simulink model "cooling_model"  (R2022a)
settings: Solver=VariableStepAuto  StartTime=4192  StopTime=20000  RelTol=1e-3
values from neighbouring files (symbols this model uses):
  area_air_fan = (fan_qty*pi.*fan_dia^2)./4'    [Cooling_Script.m]
  area_fins = n_fins * (h_fin-delta_fin) * w_radiator * 2    [Cooling_Script.m]
  area_fins_inverter = n_fins_inverter * (h_fin_inverter-delta_fin_inverter) * w_radiator_inverter * 2    [Cooling_Script.m]
  area_fins_motor = n_fins_motor * (h_fin_motor-delta_fin_motor) * w_radiator_motor * 2    [Cooling_Script.m]
  area_primary = 2 * L_tube * w_radiator * (n_fin_rows) - 2 * delta_fin * w_radiator * n_fins + 2 * h_fin * w_radiator * n_fin_rows + 2 * h_tube * n_tubes * L_tube    [Cooling_Script.m]
  area_primary_inverter = 2 * L_tube_inverter * w_radiator_inverter * (n_fin_rows_inverter) - 2 * delta_fin_inverter * w_radiator_inverter * n_fins_inverter + 2 * h_fin_inverter * w_radiator_inverter * n_fin_rows_inverter + 2 * h_tube_inverter * n_tubes_inverter * L_tube_inverter    [Cooling_Script.m]
  area_primary_motor = 2 * L_tube_motor * w_radiator_motor * (n_fin_rows_motor) - 2 * delta_fin_motor * w_radiator_motor * n_fins_motor + 2 * h_fin_motor * w_radiator_motor * n_fin_rows_motor + 2 * h_tube_motor * n_tubes_motor * L_tube_motor    [Cooling_Script.m]
  cp_air = 1004    [Cooling_Script.m]
  h_tube = 0.0015    [Cooling_Script.m]
  h_tube_inverter = 0.0015    [Cooling_Script.m]
  h_tube_motor = 0.0015    [Cooling_Script.m]
  HC_min = 10    [Cooling_Script.m]
  HC_nom = 100    [Cooling_Script.m]
  L_tube = 46*25.4./1000    [Cooling_Script.m]
  L_tube_inverter = 46*25.4./1000    [Cooling_Script.m]
  L_tube_motor = 46*25.4./1000    [Cooling_Script.m]
  n_tubes = 36    [Cooling_Script.m]
  n_tubes_inverter = 36    [Cooling_Script.m]
  n_tubes_motor = 36    [Cooling_Script.m]
  rho_air = 1.2    [Cooling_Script.m]
  vel_air_nom = 1    [Cooling_Script.m]
  w_radiator = 2.6*25.4    (= 66.04)    [Cooling_Script.m]
  w_radiator_inverter = 2.6*25.4    (= 66.04)    [Cooling_Script.m]
  w_radiator_motor = 2.6*25.4    (= 66.04)    [Cooling_Script.m]
libraries: fl_lib x65, nesl_utility x35, SimscapeFluids_lib x12, aerolibconvert2 x9
(part 1 of 2)
settings Model: PacingRate=7  Creator=saumilj  LastModifiedBy=saumilj

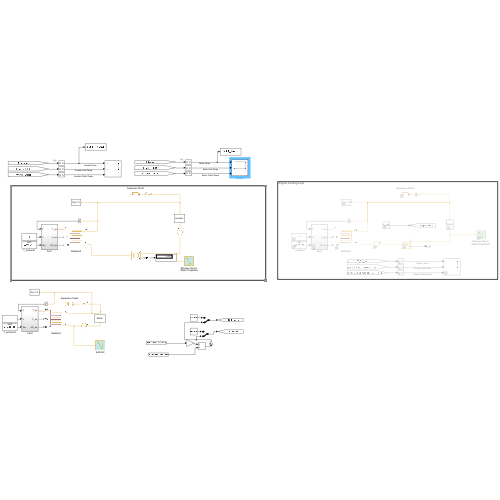
[thumbnail: Simulink's stored preview of the top-level diagram]
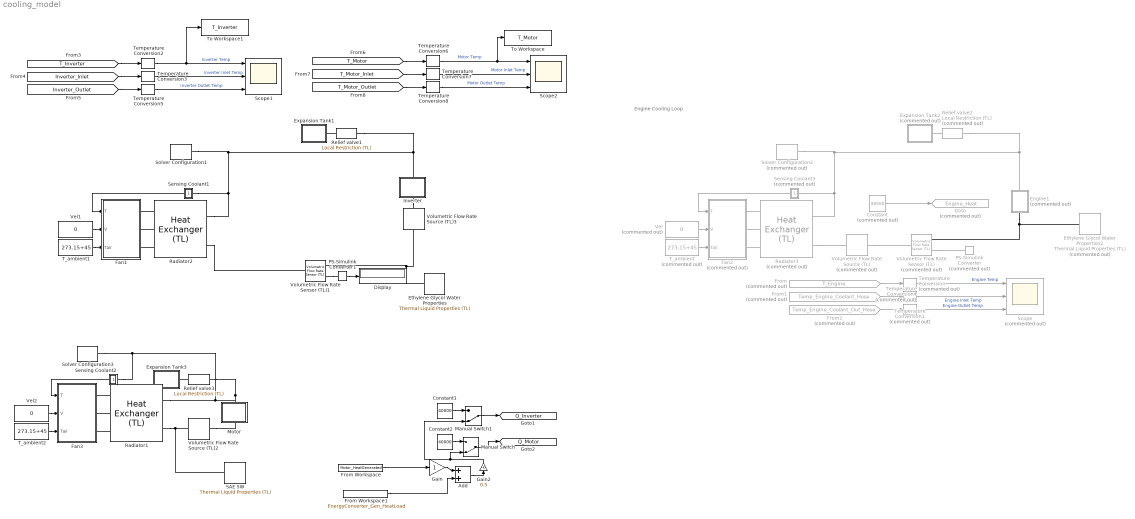
== system cooling_model ==
  note: Engine Cooling Loop
  Add : Sum
  Constant : Constant  Commented=on  Value=80000
  Constant1 : Constant  Value=40000
  Constant2 : Constant  Value=40000
  Display : Display
  Engine1 : Subsystem  Tag=PublishSubsystem  Commented=on
      settings: PortSchema="{\"entries\":[{\"content\":{\"sides\":[{\"content\":{\"connectorIds\":[]},\"type\":\"ConnectorPlacement.EquallySpacedRectSide\",\"uuid\":\"ac213905-571d-4802-86f4-209dcc725585\"},{\"content\":{\"connectorIds\":[],\"side\":\"RIGHT\"},\"type\":\"ConnectorPlacement.EquallySpacedRectSide\",\"uuid\":\"d2c48898-fea5-4b13-99f1-692c4ae7991e\"},{\"content\":{\"connectorIds\":[\"LConn1\"],\"side\":\"TOP\"},\"type\":\"ConnectorPlacement.EquallySpacedRectSide\",\"uuid\":\"96c2b262-82b5-4793-b4c5-6a92a22b5fd9\"},{\"content\":{\"connectorIds\":[\"RConn1\"],\"side\":\"BOTTOM\"},\"type\":\"ConnectorPlacement.EquallySpacedRectSide\",\"uuid\":\"b403586d-fe60-4930-b0ca-7a9e68811f94\"}]},\"type\":\"ConnectorPlacement.EquallySpacedConnector\",\"uuid\":\"afb30120-f19b-44b2-997c-30915d066b29\"}],\"packageUris\":[\"http://schema.mathworks.com/mf0/Connector/R2020b\"],\"version\":\"1.0\"}"
      mask Display: disp(get_param(gcb, 'Name'))
  Ethylene Glycol Water Properties : SimscapeFluids_lib/Thermal Liquid/Utilities/Thermal Liquid Properties (TL)  fluid_list=3  concentration_param_EG=1  concentration_param_PG=1  c_mass_SW=3.5e-3  c_mass_EG=0.1  c_mass_PG=0.1  c_mass_GL=0.1  c_vol_EG=0.5  c_vol_PG=0.1  beta_const_EG=2.1791 GPa  beta_const_PG=2.1791 GPa  beta_const_GL=2.1791 GPa  p_min_EG=0.01 MPa  p_min_PG=0.01 MPa  p_min_GL=0.01 MPa  p_max_EG=50 MPa  p_max_PG=50 MPa  p_max_GL=50 MPa  p_atm=0.101325 MPa
      settings: SourceProductBaseCode=SH
  Ethylene Glycol Water Properties2 : SimscapeFluids_lib/Thermal Liquid/Utilities/Thermal Liquid Properties (TL)  Commented=on  fluid_list=3  concentration_param_EG=1  concentration_param_PG=1  c_mass_SW=3.5e-3  c_mass_EG=0.1  c_mass_PG=0.1  c_mass_GL=0.1  c_vol_EG=0.5  c_vol_PG=0.1  beta_const_EG=2.1791 GPa  beta_const_PG=2.1791 GPa  beta_const_GL=2.1791 GPa  p_min_EG=0.01 MPa  p_min_PG=0.01 MPa  p_min_GL=0.01 MPa  p_max_EG=50 MPa  p_max_PG=50 MPa  p_max_GL=50 MPa  p_atm=0.101325 MPa
      settings: SourceProductBaseCode=SH
  Expansion Tank1 : Subsystem
      mask Display: image('sscfluids_engine_cooling_system_expansion_tank_image.png')
  Expansion Tank2 : Subsystem  Commented=on
      mask Display: image('sscfluids_engine_cooling_system_expansion_tank_image.png')
  Expansion Tank3 : Subsystem
      mask Display: image('sscfluids_engine_cooling_system_expansion_tank_image.png')
  Fan1 : Subsystem
  Fan2 : Subsystem  Commented=on
  Fan3 : Subsystem
  From : From  Commented=on  GotoTag=T_Engine  TagVisibility=global
  From Workspace : FromWorkspace  VariableName=Motor_HeatGenerated
  From Workspace1 : FromWorkspace  VariableName=EnergyConverter_Gen_HeatLoad
  From1 : From  Commented=on  GotoTag=Temp_Engine_Coolant_Hose  TagVisibility=global
  From2 : From  Commented=on  GotoTag=Temp_Engine_Coolant_Out_Hose  TagVisibility=global
  Gain : Gain
  Gain2 : Gain  Gain=0.5
  Goto : Goto  Commented=on  GotoTag=Engine_Heat  TagVisibility=global
  Inverter : Subsystem  Tag=PublishSubsystem
      settings: PortSchema="{\"entries\":[{\"content\":{\"sides\":[{\"content\":{\"connectorIds\":[]},\"type\":\"ConnectorPlacement.EquallySpacedRectSide\",\"uuid\":\"ac213905-571d-4802-86f4-209dcc725585\"},{\"content\":{\"connectorIds\":[],\"side\":\"RIGHT\"},\"type\":\"ConnectorPlacement.EquallySpacedRectSide\",\"uuid\":\"d2c48898-fea5-4b13-99f1-692c4ae7991e\"},{\"content\":{\"connectorIds\":[\"LConn1\"],\"side\":\"TOP\"},\"type\":\"ConnectorPlacement.EquallySpacedRectSide\",\"uuid\":\"96c2b262-82b5-4793-b4c5-6a92a22b5fd9\"},{\"content\":{\"connectorIds\":[\"RConn1\"],\"side\":\"BOTTOM\"},\"type\":\"ConnectorPlacement.EquallySpacedRectSide\",\"uuid\":\"b403586d-fe60-4930-b0ca-7a9e68811f94\"}]},\"type\":\"ConnectorPlacement.EquallySpacedConnector\",\"uuid\":\"afb30120-f19b-44b2-997c-30915d066b29\"}],\"packageUris\":[\"http://schema.mathworks.com/mf0/Connector/R2020b\"],\"version\":\"1.0\"}"
      mask Display: disp(get_param(gcb, 'Name'))
  Manual Switch : ManualSwitch  CurrentSetting=0
  Manual Switch1 : ManualSwitch  CurrentSetting=0
  Motor : Subsystem  Tag=PublishSubsystem
      settings: PortSchema="{\"entries\":[{\"content\":{\"sides\":[{\"content\":{\"connectorIds\":[]},\"type\":\"ConnectorPlacement.EquallySpacedRectSide\",\"uuid\":\"ac213905-571d-4802-86f4-209dcc725585\"},{\"content\":{\"connectorIds\":[],\"side\":\"RIGHT\"},\"type\":\"ConnectorPlacement.EquallySpacedRectSide\",\"uuid\":\"d2c48898-fea5-4b13-99f1-692c4ae7991e\"},{\"content\":{\"connectorIds\":[\"LConn1\"],\"side\":\"TOP\"},\"type\":\"ConnectorPlacement.EquallySpacedRectSide\",\"uuid\":\"96c2b262-82b5-4793-b4c5-6a92a22b5fd9\"},{\"content\":{\"connectorIds\":[\"RConn1\"],\"side\":\"BOTTOM\"},\"type\":\"ConnectorPlacement.EquallySpacedRectSide\",\"uuid\":\"b403586d-fe60-4930-b0ca-7a9e68811f94\"}]},\"type\":\"ConnectorPlacement.EquallySpacedConnector\",\"uuid\":\"afb30120-f19b-44b2-997c-30915d066b29\"}],\"packageUris\":[\"http://schema.mathworks.com/mf0/Connector/R2020b\"],\"version\":\"1.0\"}"
      mask Display: disp(get_param(gcb, 'Name'))
  PS-Simulink Converter : nesl_utility/PS-Simulink Converter  Commented=on  PhysicalDomain=network_engine_domain  SubClassName=ps_output  LeftPortType=input  RightPortType=output  PseudoPeriodic=off  Frequencies=[]  VectorFormat=inherit  Unit=inherit  AffineConversion=off
      settings: SourceProductBaseCode=SS,PW,VE
  PS-Simulink Converter1 : nesl_utility/PS-Simulink Converter  PhysicalDomain=network_engine_domain  SubClassName=ps_output  LeftPortType=input  RightPortType=output  PseudoPeriodic=off  Frequencies=[]  VectorFormat=inherit  Unit=inherit  AffineConversion=off
      settings: SourceProductBaseCode=SS,PW,VE
  Radiator1 : SimscapeFluids_lib/Fluid Network Interfaces/Heat Exchangers/Heat Exchanger (TL)  hex_type=fluids.interfaces.enum.flow_arrangement_spec.parallel_counter  shell_num=1  cross_type=4  NTU_TLU=[0.5, 1.0, 2.0, 3.0, 4.0, 5.0]  CR_TLU=[0.0, 0.25, 0.5, 0.75, 1.0]  eff_TLU=[0.3, 0.3, 0.3, 0.3, 0.3; 0.6, 0.55, 0.5, 0.47, 0.43; 0.85, 0.76, 0.68, 0.61, 0.55; 0.94, 0.83, 0.72, 0.65, 0.58; 0.98, 0.86, 0.75, 0.66, 0.58; 0.99, 0.86, 0.75, 0.66, 0.58]  R_wall=0.014/(381*n_tubes_motor*w_radiator_motor*L_tube_motor) K/W  min_flow_area_1=n_tubes_motor*(w_radiator_motor*h_tube_motor) m^2  Dh_press_1=4*(w_radiator_motor*h_tube_motor)/(2 * (w_radiator_motor+h_tube_motor)) m  liquid_volume_1=n_tubes_motor*(w_radiator_motor*h_tube_motor)*L_tube_motor m^3  Re_lam_1=2000  Re_tur_1=4000  pressure_loss_spec_1=2  pressure_loss_coeff_1=15  length_press_1=L_tube_motor m  length_add_1=0.1 m  roughness_1=15e-6 m  Re_friction_TLU_1=[400.0, 1000.0, 1500.0, 3000.0, 4000.0, 6000.0, 10000.0, 20000.0, 40000.0, 60000.0, 100000.0, 100000000.0]  friction_factor_TLU_1=[0.264, 0.112, 0.071, 0.0417, 0.0387, 0.0268, 0.025, 0.0232, 0.0226, 0.022, 0.0214, 0.0214]  shape_factor_1=64  Re_Euler_TLU_1=[50.0, 500.0, 1000.0, 2000.0]  Euler_TLU_1=[4.4505, 0.6864, 0.4791, 0.3755]  heat_transfer_spec_1=2  heat_transfer_area_1=n_tubes_motor*2*(L_tube_motor*w_radiator_motor+L_tube_motor*h_tube_motor) m^2  heat_coeff_1=2000 W/(m^2 * K)  length_heat_1=L_tube_motor m  Nu_lam_1=3.66  Re_Colburn_TLU_1=[100.0, 150.0, 1000.0]  Colburn_factor_TLU_1=[0.019, 0.013, 0.002]  Re_Nu_TLU_1=[100.0, 150.0, 1000.0]  Pr_Nu_TLU_1=[1.0, 10.0]  Nu_TLU_1=[3.72, 4.21; 3.75, 4.44; 4.21, 7.15]  fouling_factor_1=0 m^2*K/W  min_heat_coeff_1=5 W/(m^2 * K)  heat_transfer_area_2=area_primary_motor+area_fins_motor m^2  fouling_factor_2=0 m^2*K/W  min_heat_coeff_2=0.01 W/(m^2 * K)  dynamic_compressibility_1=1  T0_1=293.15+25 K  p0_1=0.101325 MPa  mdot1_TLU=[.1, .2] kg/s  mdot2_TLU=[.2, .3] kg/s  SD_TLU=[35, 35; 50, 50] kW/K  Q_check=1  mdot_dp_TLU_1=[.1, .2] kg/s  p_diff_TLU_1=[.003, .005] MPa  T_ref_in_1=293.15 K  p_ref_in_1=0.101325 MPa  mdot_threshold_1=1e-3 kg/s  area_1=0.01 m^2
      settings: SourceProductBaseCode=SH  InternalSimscapePortConfiguration="{\"Bottom\":[],\"Left\":[{\"id\":\"A1\",\"label\":\"A1\",\"type\":\"foundation.thermal_liquid.thermal_liquid\"},{\"id\":\"B1\",\"label\":\"B1\",\"type\":\"foundation.thermal_liquid.thermal_liquid\"}],\"Right\":[{\"id\":\"H2\",\"label\":\"H2\",\"type\":\"foundation.thermal.thermal\"},{\"id\":\"C2\",\"label\":\"C2\",\"type\":\"input\"},{\"id\":\"HC2\",\"label\":\"HC2\",\"type\":\"input\"}],\"Top\":[]}"
  Radiator2 : SimscapeFluids_lib/Fluid Network Interfaces/Heat Exchangers/Heat Exchanger (TL)  hex_type=fluids.interfaces.enum.flow_arrangement_spec.parallel_counter  shell_num=1  cross_type=4  NTU_TLU=[0.5, 1.0, 2.0, 3.0, 4.0, 5.0]  CR_TLU=[0.0, 0.25, 0.5, 0.75, 1.0]  eff_TLU=[0.3, 0.3, 0.3, 0.3, 0.3; 0.6, 0.55, 0.5, 0.47, 0.43; 0.85, 0.76, 0.68, 0.61, 0.55; 0.94, 0.83, 0.72, 0.65, 0.58; 0.98, 0.86, 0.75, 0.66, 0.58; 0.99, 0.86, 0.75, 0.66, 0.58]  R_wall=0.014/(381*n_tubes_inverter*w_radiator_inverter*L_tube_inverter) K/W  min_flow_area_1=n_tubes_inverter*(w_radiator_inverter*h_tube_inverter) m^2  Dh_press_1=4*(w_radiator_inverter*h_tube_inverter)/(2 * (w_radiator_inverter+h_tube_inverter)) m  liquid_volume_1=n_tubes_inverter*(w_radiator_inverter*h_tube_inverter)*L_tube_inverter m^3  Re_lam_1=2000  Re_tur_1=4000  pressure_loss_spec_1=2  pressure_loss_coeff_1=15  length_press_1=L_tube_inverter m  length_add_1=0.1 m  roughness_1=15e-6 m  Re_friction_TLU_1=[400.0, 1000.0, 1500.0, 3000.0, 4000.0, 6000.0, 10000.0, 20000.0, 40000.0, 60000.0, 100000.0, 100000000.0]  friction_factor_TLU_1=[0.264, 0.112, 0.071, 0.0417, 0.0387, 0.0268, 0.025, 0.0232, 0.0226, 0.022, 0.0214, 0.0214]  shape_factor_1=64  Re_Euler_TLU_1=[50.0, 500.0, 1000.0, 2000.0]  Euler_TLU_1=[4.4505, 0.6864, 0.4791, 0.3755]  heat_transfer_spec_1=2  heat_transfer_area_1=n_tubes_inverter*2*(L_tube_inverter*w_radiator_inverter+L_tube_inverter*h_tube_inverter) m^2  heat_coeff_1=2000 W/(m^2 * K)  length_heat_1=L_tube_inverter m  Nu_lam_1=3.66  Re_Colburn_TLU_1=[100.0, 150.0, 1000.0]  Colburn_factor_TLU_1=[0.019, 0.013, 0.002]  Re_Nu_TLU_1=[100.0, 150.0, 1000.0]  Pr_Nu_TLU_1=[1.0, 10.0]  Nu_TLU_1=[3.72, 4.21; 3.75, 4.44; 4.21, 7.15]  fouling_factor_1=0 m^2*K/W  min_heat_coeff_1=5 W/(m^2 * K)  heat_transfer_area_2=area_primary_inverter+area_fins_inverter m^2  fouling_factor_2=0 m^2*K/W  min_heat_coeff_2=0.01 W/(m^2 * K)  dynamic_compressibility_1=1  T0_1=293.15+25 K  p0_1=0.101325 MPa  mdot1_TLU=[.1, .2] kg/s  mdot2_TLU=[.2, .3] kg/s  SD_TLU=[35, 35; 50, 50] kW/K  Q_check=1  mdot_dp_TLU_1=[.1, .2] kg/s  p_diff_TLU_1=[.003, .005] MPa  T_ref_in_1=293.15 K  p_ref_in_1=0.101325 MPa  mdot_threshold_1=1e-3 kg/s  area_1=0.01 m^2
      settings: SourceProductBaseCode=SH  InternalSimscapePortConfiguration="{\"Bottom\":[],\"Left\":[{\"id\":\"A1\",\"label\":\"A1\",\"type\":\"foundation.thermal_liquid.thermal_liquid\"},{\"id\":\"B1\",\"label\":\"B1\",\"type\":\"foundation.thermal_liquid.thermal_liquid\"}],\"Right\":[{\"id\":\"H2\",\"label\":\"H2\",\"type\":\"foundation.thermal.thermal\"},{\"id\":\"C2\",\"label\":\"C2\",\"type\":\"input\"},{\"id\":\"HC2\",\"label\":\"HC2\",\"type\":\"input\"}],\"Top\":[]}"
  Radiator3 : SimscapeFluids_lib/Fluid Network Interfaces/Heat Exchangers/Heat Exchanger (TL)  Commented=on  hex_type=fluids.interfaces.enum.flow_arrangement_spec.parallel_counter  shell_num=1  cross_type=4  NTU_TLU=[0.5, 1.0, 2.0, 3.0, 4.0, 5.0]  CR_TLU=[0.0, 0.25, 0.5, 0.75, 1.0]  eff_TLU=[0.3, 0.3, 0.3, 0.3, 0.3; 0.6, 0.55, 0.5, 0.47, 0.43; 0.85, 0.76, 0.68, 0.61, 0.55; 0.94, 0.83, 0.72, 0.65, 0.58; 0.98, 0.86, 0.75, 0.66, 0.58; 0.99, 0.86, 0.75, 0.66, 0.58]  R_wall=0.014/(381*n_tubes*w_radiator*L_tube) K/W  min_flow_area_1=n_tubes*(w_radiator*h_tube) m^2  Dh_press_1=4*(w_radiator*h_tube)/(2 * (w_radiator+h_tube)) m  liquid_volume_1=n_tubes*(w_radiator*h_tube)*L_tube m^3  Re_lam_1=2000  Re_tur_1=4000  pressure_loss_spec_1=2  pressure_loss_coeff_1=15  length_press_1=L_tube m  length_add_1=0.1 m  roughness_1=15e-6 m  Re_friction_TLU_1=[400.0, 1000.0, 1500.0, 3000.0, 4000.0, 6000.0, 10000.0, 20000.0, 40000.0, 60000.0, 100000.0, 100000000.0]  friction_factor_TLU_1=[0.264, 0.112, 0.071, 0.0417, 0.0387, 0.0268, 0.025, 0.0232, 0.0226, 0.022, 0.0214, 0.0214]  shape_factor_1=64  Re_Euler_TLU_1=[50.0, 500.0, 1000.0, 2000.0]  Euler_TLU_1=[4.4505, 0.6864, 0.4791, 0.3755]  heat_transfer_spec_1=2  heat_transfer_area_1=n_tubes*2*(L_tube*w_radiator+L_tube*h_tube) m^2  heat_coeff_1=2000 W/(m^2 * K)  length_heat_1=L_tube m  Nu_lam_1=3.66  Re_Colburn_TLU_1=[100.0, 150.0, 1000.0]  Colburn_factor_TLU_1=[0.019, 0.013, 0.002]  Re_Nu_TLU_1=[100.0, 150.0, 1000.0]  Pr_Nu_TLU_1=[1.0, 10.0]  Nu_TLU_1=[3.72, 4.21; 3.75, 4.44; 4.21, 7.15]  fouling_factor_1=0 m^2*K/W  min_heat_coeff_1=5 W/(m^2 * K)  heat_transfer_area_2=area_primary+area_fins m^2  fouling_factor_2=0 m^2*K/W  min_heat_coeff_2=0.01 W/(m^2 * K)  dynamic_compressibility_1=1  T0_1=293.15 K  p0_1=0.101325 MPa  mdot1_TLU=[.1, .2] kg/s  mdot2_TLU=[.2, .3] kg/s  SD_TLU=[35, 35; 50, 50] kW/K  Q_check=1  mdot_dp_TLU_1=[.1, .2] kg/s  p_diff_TLU_1=[.003, .005] MPa  T_ref_in_1=293.15 K  p_ref_in_1=0.101325 MPa  mdot_threshold_1=1e-3 kg/s  area_1=0.01 m^2
      settings: SourceProductBaseCode=SH  InternalSimscapePortConfiguration="{\"Bottom\":[],\"Left\":[{\"id\":\"A1\",\"label\":\"A1\",\"type\":\"foundation.thermal_liquid.thermal_liquid\"},{\"id\":\"B1\",\"label\":\"B1\",\"type\":\"foundation.thermal_liquid.thermal_liquid\"}],\"Right\":[{\"id\":\"H2\",\"label\":\"H2\",\"type\":\"foundation.thermal.thermal\"},{\"id\":\"C2\",\"label\":\"C2\",\"type\":\"input\"},{\"id\":\"HC2\",\"label\":\"HC2\",\"type\":\"input\"}],\"Top\":[]}"
  Relief valve1 : fl_lib/Thermal Liquid/Elements/Local Restriction (TL)  restriction_type=foundation.enum.restriction_type.fixed  restriction_area=pi*0.005^2 m^2  min_area=1e-10 m^2  max_area=0.005 m^2  area=pi*0.01^2 m^2  Cd=0.7  pressure_recovery=1  Re_c=12
      settings: SourceProductBaseCode=PW,SS,VE
  Relief valve2 : fl_lib/Thermal Liquid/Elements/Local Restriction (TL)  Commented=on  restriction_type=foundation.enum.restriction_type.fixed  restriction_area=pi*0.005^2 m^2  min_area=1e-10 m^2  max_area=0.005 m^2  area=pi*0.01^2 m^2  Cd=0.7  pressure_recovery=1  Re_c=12
      settings: SourceProductBaseCode=PW,SS,VE
  Relief valve3 : fl_lib/Thermal Liquid/Elements/Local Restriction (TL)  restriction_type=foundation.enum.restriction_type.fixed  restriction_area=pi*0.005^2 m^2  min_area=1e-10 m^2  max_area=0.005 m^2  area=pi*0.01^2 m^2  Cd=0.7  pressure_recovery=1  Re_c=12
      settings: SourceProductBaseCode=PW,SS,VE
  SAE 5W : SimscapeFluids_lib/Thermal Liquid/Utilities/Thermal Liquid Properties (TL)  fluid_list=fluids.thermal_liquid.utilities.enum.thermal_liquid_fluid_list.sae5w30  concentration_param_EG=1  concentration_param_PG=1  c_mass_SW=3.5e-3  c_mass_EG=0.1  c_mass_PG=0.1  c_mass_GL=0.1  c_vol_EG=0.5  c_vol_PG=0.1  beta_const_EG=2.1791 GPa  beta_const_PG=2.1791 GPa  beta_const_GL=2.1791 GPa  p_min_EG=0.01 MPa  p_min_PG=0.01 MPa  p_min_GL=0.01 MPa  p_max_EG=50 MPa  p_max_PG=50 MPa  p_max_GL=50 MPa  p_atm=0.101325 MPa
      settings: SourceProductBaseCode=SH
  Scope : Scope  Commented=on  NumInputPorts=3
  Scope1 : Scope  NumInputPorts=3
  Scope2 : Scope  NumInputPorts=3
  Sensing Coolant1 : Subsystem
      mask Display: disp('T');
  Sensing Coolant2 : Subsystem
      mask Display: disp('T');
  Sensing Coolant3 : Subsystem  Commented=on
      mask Display: disp('T');
  Solver Configuration1 : nesl_utility/Solver Configuration  PhysicalDomain=network_engine_domain  SubClassName=solver  LeftPortType=input  RightPortType=generic  Tones=[]  Harmonics=[]  SimulateNoise=off  Profile=off  UseLocalSampling=off  EnableSwitchedLinearOptims=on  FrequencyDomain=off  UseCCode=off  RelTol=0.001  AbsTol=1e-06  MinStep=1e-09  ToWorkspace=off  RevertToSquareIcSolve=off  NumHomotopyIterations=100  PhasorMode=off  PhasorModeNumHarmonics=1  IndexReductionMethod=DerivativeReplacement  DoDC=off  ResidualTolerance=1e-09  UseLocalSolver=off  LocalSolverChoice=NE_BACKWARD_EULER_ADVANCER  LocalSolverSampleTime=0.001  DoFixedCost=off  MaxNonlinIter=3  MaxModeIter=2  ComputeImpulses=off  ImpulseIterations=2  LinearAlgebra=auto  LinearAlgebraNumThread=0  EquationFormulation=NE_TIME_EF  DelaysMemoryBudget=1024  AutomaticFiltering=on  FilteringTimeConstant=0.001  PartitionStorageMethod=AS_NEEDED  PartitionMemoryBudget=1024  PartitionMethod=ROBUST
      settings: SourceProductBaseCode=SS,PW,VE
  Solver Configuration2 : nesl_utility/Solver Configuration  Commented=on  PhysicalDomain=network_engine_domain  SubClassName=solver  LeftPortType=input  RightPortType=generic  Tones=[]  Harmonics=[]  SimulateNoise=off  Profile=off  UseLocalSampling=off  EnableSwitchedLinearOptims=on  FrequencyDomain=off  UseCCode=off  RelTol=0.001  AbsTol=1e-06  MinStep=1e-09  ToWorkspace=off  RevertToSquareIcSolve=off  NumHomotopyIterations=100  PhasorMode=off  PhasorModeNumHarmonics=1  IndexReductionMethod=DerivativeReplacement  DoDC=off  ResidualTolerance=1e-09  UseLocalSolver=off  LocalSolverChoice=NE_BACKWARD_EULER_ADVANCER  LocalSolverSampleTime=0.001  DoFixedCost=off  MaxNonlinIter=3  MaxModeIter=2  ComputeImpulses=off  ImpulseIterations=2  LinearAlgebra=auto  LinearAlgebraNumThread=0  EquationFormulation=NE_TIME_EF  DelaysMemoryBudget=1024  AutomaticFiltering=on  FilteringTimeConstant=0.001  PartitionStorageMethod=AS_NEEDED  PartitionMemoryBudget=1024  PartitionMethod=ROBUST
      settings: SourceProductBaseCode=SS,PW,VE
  Solver Configuration3 : nesl_utility/Solver Configuration  PhysicalDomain=network_engine_domain  SubClassName=solver  LeftPortType=input  RightPortType=generic  Tones=[]  Harmonics=[]  SimulateNoise=off  Profile=off  UseLocalSampling=off  EnableSwitchedLinearOptims=on  FrequencyDomain=off  UseCCode=off  RelTol=0.001  AbsTol=1e-06  MinStep=1e-09  ToWorkspace=off  RevertToSquareIcSolve=off  NumHomotopyIterations=100  PhasorMode=off  PhasorModeNumHarmonics=1  IndexReductionMethod=DerivativeReplacement  DoDC=off  ResidualTolerance=1e-09  UseLocalSolver=off  LocalSolverChoice=NE_BACKWARD_EULER_ADVANCER  LocalSolverSampleTime=0.001  DoFixedCost=off  MaxNonlinIter=3  MaxModeIter=2  ComputeImpulses=off  ImpulseIterations=2  LinearAlgebra=auto  LinearAlgebraNumThread=0  EquationFormulation=NE_TIME_EF  DelaysMemoryBudget=1024  AutomaticFiltering=on  FilteringTimeConstant=0.001  PartitionStorageMethod=AS_NEEDED  PartitionMemoryBudget=1024  PartitionMethod=ROBUST
      settings: SourceProductBaseCode=SS,PW,VE
  T_ambient : Constant  Commented=on  Value=273.15+45
  T_ambient1 : Constant  Value=273.15+45
  T_ambient2 : Constant  Value=273.15+45
  Temperature Conversion : aerolibconvert2/Temperature Conversion  Commented=on  IU=K  OU=C
      settings: SourceProductBaseCode=AE
  Temperature Conversion1 : aerolibconvert2/Temperature Conversion  Commented=on  IU=K  OU=C
      settings: SourceProductBaseCode=AE
  Temperature Conversion{2..3,5..8} (6 alike) : aerolibconvert2/Temperature Conversion  IU=K  OU=C
      settings: SourceProductBaseCode=AE
  Temperature Conversion4 : aerolibconvert2/Temperature Conversion  Commented=on  IU=K  OU=C
      settings: SourceProductBaseCode=AE
  To Workspace : ToWorkspace  VariableName=T_Motor  SaveFormat=Timeseries  SampleTime=-1
  To Workspace1 : ToWorkspace  VariableName=T_Inverter  SaveFormat=Timeseries  SampleTime=-1
  Vel : Constant  Commented=on  Value=0
  Vel1 : Constant  Value=0
  Vel2 : Constant  Value=0
  Volumetric Flow Rate Sensor (TL) : fl_lib/Thermal Liquid/Sensors/Volumetric Flow Rate Sensor (TL)  Commented=on
      settings: SourceProductBaseCode=PW,SS,VE  InternalSimscapePortConfiguration="{\"Bottom\":[],\"Left\":[{\"id\":\"A\",\"label\":\"A\",\"type\":\"foundation.thermal_liquid.thermal_liquid\"}],\"Right\":[{\"id\":\"B\",\"label\":\"B\",\"type\":\"foundation.thermal_liquid.thermal_liquid\"},{\"id\":\"V\",\"label\":\"V\",\"type\":\"output\"}],\"Top\":[]}"
  Volumetric Flow Rate Sensor (TL)1 : fl_lib/Thermal Liquid/Sensors/Volumetric Flow Rate Sensor (TL)
      settings: SourceProductBaseCode=PW,SS,VE  InternalSimscapePortConfiguration="{\"Bottom\":[],\"Left\":[{\"id\":\"A\",\"label\":\"A\",\"type\":\"foundation.thermal_liquid.thermal_liquid\"}],\"Right\":[{\"id\":\"B\",\"label\":\"B\",\"type\":\"foundation.thermal_liquid.thermal_liquid\"},{\"id\":\"V\",\"label\":\"V\",\"type\":\"output\"}],\"Top\":[]}"
  Volumetric Flow Rate Source (TL) : fl_lib/Thermal Liquid/Sources/Volumetric Flow Rate Source (TL)  Commented=on  commanded_volumetric_flow=60 lpm  area=0.01 m^2
      settings: SourceProductBaseCode=PW,SS,VE  InternalSimscapePortConfiguration="{\"Bottom\":[],\"Left\":[{\"id\":\"A\",\"label\":\"A\",\"type\":\"foundation.thermal_liquid.thermal_liquid\"}],\"Right\":[{\"id\":\"B\",\"label\":\"B\",\"type\":\"foundation.thermal_liquid.thermal_liquid\"}],\"Top\":[]}"
  Volumetric Flow Rate Source (TL)2 : fl_lib/Thermal Liquid/Sources/Volumetric Flow Rate Source (TL)  commanded_volumetric_flow=20*6 lpm  area=0.01 m^2
      settings: SourceProductBaseCode=PW,SS,VE  InternalSimscapePortConfiguration="{\"Bottom\":[],\"Left\":[{\"id\":\"A\",\"label\":\"A\",\"type\":\"foundation.thermal_liquid.thermal_liquid\"}],\"Right\":[{\"id\":\"B\",\"label\":\"B\",\"type\":\"foundation.thermal_liquid.thermal_liquid\"}],\"Top\":[]}"
  Volumetric Flow Rate Source (TL)3 : fl_lib/Thermal Liquid/Sources/Volumetric Flow Rate Source (TL)  commanded_volumetric_flow=60 lpm  area=0.01 m^2
      settings: SourceProductBaseCode=PW,SS,VE  InternalSimscapePortConfiguration="{\"Bottom\":[],\"Left\":[{\"id\":\"A\",\"label\":\"A\",\"type\":\"foundation.thermal_liquid.thermal_liquid\"}],\"Right\":[{\"id\":\"B\",\"label\":\"B\",\"type\":\"foundation.thermal_liquid.thermal_liquid\"}],\"Top\":[]}"
  tag scope: Q_Inverter=global, Q_Motor=global
  wires:
  Constant/1 -> Goto/1
  Sensing Coolant3/1(Out1) -> Fan2/1(T)
  T_ambient/1 -> Fan2/3(Tair)
  Vel/1 -> Fan2/2(V)
  From/1 -> Temperature Conversion/1
  From1/1 -> Temperature Conversion1/1
  From2/1 -> Temperature Conversion4/1
  Temperature Conversion/1 -> Scope/1  "Engine Temp"
  Temperature Conversion1/1 -> Scope/2  "Engine Inlet Temp"
  Temperature Conversion4/1 -> Scope/3  "Engine Outlet Temp"
  Temperature Conversion5/1 -> Scope1/3  "Inverter Outlet Temp"
  Temperature Conversion3/1 -> Scope1/2  "Inverter Inlet Temp"
  Temperature Conversion2/1 -> To Workspace1/1, Scope1/1  "Inverter Temp"
  [Inverter_Outlet] -> Temperature Conversion5/1
  [Inverter_Inlet] -> Temperature Conversion3/1
  [T_Inverter] -> Temperature Conversion2/1
  Vel1/1 -> Fan1/2(V)
  T_ambient1/1 -> Fan1/3(Tair)
  Sensing Coolant1/1(Out1) -> Fan1/1(T)
  [T_Motor] -> Temperature Conversion6/1
  [T_Motor_Inlet] -> Temperature Conversion7/1
  [T_Motor_Outlet] -> Temperature Conversion8/1
  Temperature Conversion6/1 -> To Workspace/1, Scope2/1  "Motor Temp"
  Temperature Conversion7/1 -> Scope2/2  "Motor Inlet Temp"
  Temperature Conversion8/1 -> Scope2/3  "Motor Outlet Temp"
  Constant2/1 -> Manual Switch/1
  Manual Switch/1 -> [Q_Motor]
  PS-Simulink Converter1/1 -> Display/1
  Vel2/1 -> Fan3/2(V)
  Sensing Coolant2/1(Out1) -> Fan3/1(T)
  T_ambient2/1 -> Fan3/3(Tair)
  Constant1/1 -> Manual Switch1/1
  Manual Switch1/1 -> [Q_Inverter]
  From Workspace/1 -> Gain/1
  Gain/1 -> Add/1
  From Workspace1/1 -> Add/2
  Add/1 -> Gain2/1
  Gain2/1 -> Manual Switch1/2, Manual Switch/2
  connections:
  Volumetric Flow Rate Source (TL)/RConn1 -- Volumetric Flow Rate Sensor (TL)/LConn1
  Volumetric Flow Rate Sensor (TL)/RConn2 -- PS-Simulink Converter/LConn1
  Volumetric Flow Rate Sensor (TL)/RConn1 -- Ethylene Glycol Water Properties2/RConn1 -- Engine1/RConn1
  Relief valve2/LConn1 -- Expansion Tank2/RConn1
  Radiator3/RConn1 -- Fan2/RConn1
  Radiator3/RConn2 -- Fan2/RConn2
  Radiator3/RConn3 -- Fan2/RConn3
  Solver Configuration2/RConn1 -- Engine1/LConn1 -- Relief valve2/RConn1 -- Sensing Coolant3/LConn1 -- Radiator3/LConn1
  Radiator3/LConn2 -- Volumetric Flow Rate Source (TL)/LConn1
  Inverter/LConn1 -- Relief valve1/RConn1 -- Solver Configuration1/RConn1 -- Radiator2/LConn1 -- Sensing Coolant1/LConn1
  Radiator2/RConn3 -- Fan1/RConn3
  Radiator2/RConn2 -- Fan1/RConn2
  Radiator2/RConn1 -- Fan1/RConn1
  Relief valve1/LConn1 -- Expansion Tank1/RConn1
  Radiator2/LConn2 -- Volumetric Flow Rate Sensor (TL)1/LConn1
  Ethylene Glycol Water Properties/RConn1 -- Volumetric Flow Rate Source (TL)3/LConn1 -- Volumetric Flow Rate Sensor (TL)1/RConn1
  Inverter/RConn1 -- Volumetric Flow Rate Source (TL)3/RConn1
  Volumetric Flow Rate Sensor (TL)1/RConn2 -- PS-Simulink Converter1/LConn1
  SAE 5W/RConn1 -- Radiator1/LConn2 -- Volumetric Flow Rate Source (TL)2/LConn1
  Relief valve3/RConn1 -- Radiator1/LConn1 -- Solver Configuration3/RConn1 -- Sensing Coolant2/LConn1 -- Motor/LConn1
  Volumetric Flow Rate Source (TL)2/RConn1 -- Motor/RConn1
  Relief valve3/LConn1 -- Expansion Tank3/RConn1
  Radiator1/RConn1 -- Fan3/RConn1
  Radiator1/RConn2 -- Fan3/RConn2
  Radiator1/RConn3 -- Fan3/RConn3

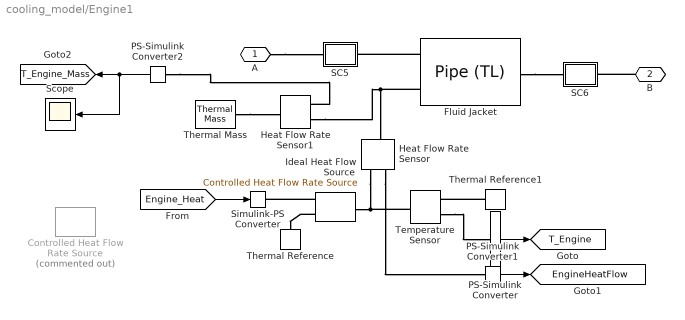
== system cooling_model/Engine1 ==
  Controlled Heat Flow Rate Source : fl_lib/Thermal/Thermal Sources/Controlled Heat Flow Rate Source  Commented=on
      settings: SourceProductBaseCode=PW,SS,VE
  Fluid Jacket : SimscapeFluids_lib/Thermal Liquid/Pipes & Fittings/Pipe (TL)  dynamic_compressibility=simscape.enum.onoff.off  inertia=simscape.enum.onoff.off  num_segments=1  pipe_length=0.2 m  area=pi*0.01^2 m^2  wall_spec=fluids.thermal_liquid.pipes_fittings.enum.wall_spec.rigid  Dh=0.005 m  wall_compliance=1.2e-6 m/MPa  wall_time_constant=0.01 s  elevation_spec=foundation.enum.constant_variable.constant  elevation_gain=0 m  g=9.81 m/s^2  pressure_loss_spec=fluids.thermal_liquid.pipes_fittings.enum.PressureLossSpec.Nominal  local_pressure_loss_spec=fluids.thermal_liquid.pipes_fittings.enum.LocalLossSpec.AggregateLength  length_add=0 m  loss_coefficient=0.1  roughness=1.5e-60 m  Re_friction_TLU=[ 400 1000 1.5e+3 3e+3 4e+3 6e+3 1e+4 2e+4 4e+4 6e+4 1e+5 1e+8 ]  friction_factor_TLU=[ 0.264 0.112 0.07099999999999999 0.0417 0.0387 0.0268 0.025 0.0232 0.0226 0.022 0.0214 0.0214 ]  shape_factor=1e-50  Re_lam=2e+3  Re_tur=4e+3  mdot_nominal=[ 0.1 1000 ] kg/s  p_diff_nominal=[ 0.00000001 0.000000001 ] MPa  mdot_threshold=1e-6 kg/s  heat_transfer_spec=fluids.thermal_liquid.pipes_fittings.enum.HeatTransferSpec.TabulatedNusselt  mdot_nominal_heat=[ 0.1 1 ] kg/s  T_in_nominal=[ 293.15 293.15 ] K  T_out_nominal=[ 300 300 ] K  p_in_nominal_heat=[ 0.101325 0.101325 ] MPa  T_wall_nominal=[ 303.15 303.15 ] K  a_coeff=0.023  b_Re_power=0.8  c_Pr_power=0.4  Nu_lam=3.66  Re_Colburn_TLU=[ 100 150 1000 ]  Colburn_factor_TLU=[ 0.019 0.013 0.002 ]  Re_Nu_TLU=Re_TLU  Pr_Nu_TLU=Pr_TLU  Nu_TLU=Nu_TLU  T0_vec=303.15 K  p0_vec=0.101325 MPa  mdot0=0.1 kg/s
      settings: SourceProductBaseCode=SH
  Heat Flow Rate Sensor : fl_lib/Thermal/Thermal Sensors/Heat Flow Rate Sensor
      settings: SourceProductBaseCode=PW,SS,VE
  Heat Flow Rate Sensor1 : fl_lib/Thermal/Thermal Sensors/Heat Flow Rate Sensor
      settings: SourceProductBaseCode=PW,SS,VE
  Ideal Heat Flow Source : fl_lib/Thermal/Thermal Sources/Controlled Heat Flow Rate Source
      settings: SourceProductBaseCode=PW,SS,VE
  PS-Simulink Converter : nesl_utility/PS-Simulink Converter  PhysicalDomain=network_engine_domain  SubClassName=ps_output  LeftPortType=input  RightPortType=output  PseudoPeriodic=off  Frequencies=[]  VectorFormat=1-D array  Unit=degC  AffineConversion=on
      settings: SourceProductBaseCode=SS,PW,VE
  PS-Simulink Converter1 : nesl_utility/PS-Simulink Converter  PhysicalDomain=network_engine_domain  SubClassName=ps_output  LeftPortType=input  RightPortType=output  PseudoPeriodic=off  Frequencies=[]  VectorFormat=inherit  Unit=inherit  AffineConversion=off
      settings: SourceProductBaseCode=SS,PW,VE
  PS-Simulink Converter2 : nesl_utility/PS-Simulink Converter  PhysicalDomain=network_engine_domain  SubClassName=ps_output  LeftPortType=input  RightPortType=output  PseudoPeriodic=off  Frequencies=[]  VectorFormat=inherit  Unit=inherit  AffineConversion=off
      settings: SourceProductBaseCode=SS,PW,VE
  SC5 : Subsystem
      mask Display: disp(get_param(gcb, 'Name'))
  SC6 : Subsystem
      mask Display: disp(get_param(gcb, 'Name'))
  Scope : Scope
  Simulink-PS Converter : nesl_utility/Simulink-PS Converter  PhysicalDomain=network_engine_domain  SubClassName=ps_input  LeftPortType=input  RightPortType=output  PseudoPeriodic=off  Frequencies=[]  NoiseDistribution=none  NoiseParameters=[]  Unit=W  AffineConversion=off  FilteringAndDerivatives=provide  SimscapeFilterOrder=1  InputFilterTimeConstant=0.001  UdotUserProvided=0
      settings: SourceProductBaseCode=SS,PW,VE
  Temperature Sensor : fl_lib/Thermal/Thermal Sensors/Temperature Sensor
      settings: SourceProductBaseCode=PW,SS,VE
  Thermal Mass : fl_lib/Thermal/Thermal Elements/Thermal Mass  mass=100 kg  sp_heat=447 J/(K*kg)  T_specify=on  T_priority=High  T=273+45 K  T_nominal_specify=off  T_nominal_unit=K  T_nominal_value=1  Q_specify=off  Q_priority=None  Q=0 W  Q_nominal_specify=off  Q_nominal_unit=W  Q_nominal_value=1
      settings: SourceProductBaseCode=PW,SS,VE
  Thermal Reference : fl_lib/Thermal/Thermal Elements/Thermal Reference
      settings: SourceProductBaseCode=PW,SS,VE
  Thermal Reference1 : fl_lib/Thermal/Thermal Elements/Thermal Reference
      settings: SourceProductBaseCode=PW,SS,VE
  A : PMIOPort  Side=Left
  B : PMIOPort  Port=2  Side=Right
  tag scope: EngineHeatFlow=global, T_Engine=global, T_Engine_Mass=global
  wires:
  [Engine_Heat] -> Simulink-PS Converter/1
  PS-Simulink Converter/1 -> [T_Engine]
  PS-Simulink Converter1/1 -> [EngineHeatFlow]
  PS-Simulink Converter2/1 -> Scope/1, [T_Engine_Mass]
  connections:
  Temperature Sensor/LConn1 -- Heat Flow Rate Sensor/RConn2 -- Ideal Heat Flow Source/LConn1
  B/RConn1 -- SC6/RConn1
  Ideal Heat Flow Source/RConn2 -- Thermal Reference/LConn1
  A/RConn1 -- SC5/LConn1
  Ideal Heat Flow Source/RConn1 -- Simulink-PS Converter/RConn1
  Thermal Reference1/LConn1 -- Temperature Sensor/RConn1
  Temperature Sensor/RConn2 -- PS-Simulink Converter/LConn1
  Fluid Jacket/LConn2 -- Heat Flow Rate Sensor1/RConn2 -- Heat Flow Rate Sensor/LConn1
  Heat Flow Rate Sensor/RConn1 -- PS-Simulink Converter1/LConn1
  Fluid Jacket/LConn1 -- SC5/RConn1
  Fluid Jacket/RConn1 -- SC6/LConn1
  PS-Simulink Converter2/LConn1 -- Heat Flow Rate Sensor1/RConn1
  Thermal Mass/LConn1 -- Heat Flow Rate Sensor1/LConn1

== system cooling_model/Expansion Tank1 ==
  Expansion Tank : SimscapeFluids_lib/Thermal Liquid/Tanks & Accumulators/Gas-Charged Accumulator (TL)  capacity=0.005 m^3  dead_volume=1e-5 m^3  p_precharge_gauge=0 MPa  k_sh=1.4  area=pi*0.01^2 m^2  stiff_coeff=1e6 MPa/m^3  damping_coeff=1e6 s*MPa/m^6  liquid_volume_specify=on  liquid_volume_priority=High  liquid_volume=1e-6 m^3  liquid_volume_nominal_specify=off  liquid_volume_nominal_unit=m^3  liquid_volume_nominal_value=1  liquid_mass_specify=off  liquid_mass_priority=None  liquid_mass=5 kg  liquid_mass_nominal_specify=off  liquid_mass_nominal_unit=kg  liquid_mass_nominal_value=1  p_accumulator_specify=off  p_accumulator_priority=High  p_accumulator=0.101325 MPa  p_accumulator_nominal_specify=off  p_accumulator_nominal_unit=MPa  p_accumulator_nominal_value=1  T_accumulator_specify=on  T_accumulator_priority=High  T_accumulator=303.15 K  T_accumulator_nominal_specify=off  T_accumulator_nominal_unit=K  T_accumulator_nominal_value=1
      settings: SourceProductBaseCode=SH  InternalSimscapePortConfiguration="{\"Bottom\":[],\"Left\":[],\"Right\":[{\"id\":\"A\",\"label\":\"A\",\"type\":\"foundation.thermal_liquid.thermal_liquid\"},{\"id\":\"H\",\"label\":\"H\",\"type\":\"foundation.thermal.thermal\"}],\"Top\":[]}"
  Perfect Insulator2 : fl_lib/Thermal/Thermal Elements/Perfect Insulator  T_specify=off  T_priority=None  T=0 K  T_nominal_specify=off  T_nominal_unit=K  T_nominal_value=1
      settings: SourceProductBaseCode=PW,SS,VE
  A : PMIOPort  Side=Right
  connections:
  Perfect Insulator2/LConn1 -- Expansion Tank/RConn2
  A/RConn1 -- Expansion Tank/RConn1

== system cooling_model/Expansion Tank2 ==
  Expansion Tank : SimscapeFluids_lib/Thermal Liquid/Tanks & Accumulators/Gas-Charged Accumulator (TL)  capacity=0.005 m^3  dead_volume=1e-5 m^3  p_precharge_gauge=0 MPa  k_sh=1.4  area=pi*0.01^2 m^2  stiff_coeff=1e6 MPa/m^3  damping_coeff=1e6 s*MPa/m^6  liquid_volume_specify=on  liquid_volume_priority=High  liquid_volume=1e-6 m^3  liquid_volume_nominal_specify=off  liquid_volume_nominal_unit=m^3  liquid_volume_nominal_value=1  liquid_mass_specify=off  liquid_mass_priority=None  liquid_mass=5 kg  liquid_mass_nominal_specify=off  liquid_mass_nominal_unit=kg  liquid_mass_nominal_value=1  p_accumulator_specify=off  p_accumulator_priority=High  p_accumulator=0.101325 MPa  p_accumulator_nominal_specify=off  p_accumulator_nominal_unit=MPa  p_accumulator_nominal_value=1  T_accumulator_specify=on  T_accumulator_priority=High  T_accumulator=303.15 K  T_accumulator_nominal_specify=off  T_accumulator_nominal_unit=K  T_accumulator_nominal_value=1
      settings: SourceProductBaseCode=SH  InternalSimscapePortConfiguration="{\"Bottom\":[],\"Left\":[],\"Right\":[{\"id\":\"A\",\"label\":\"A\",\"type\":\"foundation.thermal_liquid.thermal_liquid\"},{\"id\":\"H\",\"label\":\"H\",\"type\":\"foundation.thermal.thermal\"}],\"Top\":[]}"
  Perfect Insulator2 : fl_lib/Thermal/Thermal Elements/Perfect Insulator  T_specify=off  T_priority=None  T=0 K  T_nominal_specify=off  T_nominal_unit=K  T_nominal_value=1
      settings: SourceProductBaseCode=PW,SS,VE
  A : PMIOPort  Side=Right
  connections:
  A/RConn1 -- Expansion Tank/RConn1
  Perfect Insulator2/LConn1 -- Expansion Tank/RConn2

== system cooling_model/Expansion Tank3 ==
  Expansion Tank : SimscapeFluids_lib/Thermal Liquid/Tanks & Accumulators/Gas-Charged Accumulator (TL)  capacity=0.005 m^3  dead_volume=1e-5 m^3  p_precharge_gauge=0 MPa  k_sh=1.4  area=pi*0.01^2 m^2  stiff_coeff=1e6 MPa/m^3  damping_coeff=1e6 s*MPa/m^6  liquid_volume_specify=on  liquid_volume_priority=High  liquid_volume=1e-6 m^3  liquid_volume_nominal_specify=off  liquid_volume_nominal_unit=m^3  liquid_volume_nominal_value=1  liquid_mass_specify=off  liquid_mass_priority=None  liquid_mass=5 kg  liquid_mass_nominal_specify=off  liquid_mass_nominal_unit=kg  liquid_mass_nominal_value=1  p_accumulator_specify=off  p_accumulator_priority=High  p_accumulator=0.101325 MPa  p_accumulator_nominal_specify=off  p_accumulator_nominal_unit=MPa  p_accumulator_nominal_value=1  T_accumulator_specify=on  T_accumulator_priority=High  T_accumulator=303.15 K  T_accumulator_nominal_specify=off  T_accumulator_nominal_unit=K  T_accumulator_nominal_value=1
      settings: SourceProductBaseCode=SH  InternalSimscapePortConfiguration="{\"Bottom\":[],\"Left\":[],\"Right\":[{\"id\":\"A\",\"label\":\"A\",\"type\":\"foundation.thermal_liquid.thermal_liquid\"},{\"id\":\"H\",\"label\":\"H\",\"type\":\"foundation.thermal.thermal\"}],\"Top\":[]}"
  Perfect Insulator2 : fl_lib/Thermal/Thermal Elements/Perfect Insulator  T_specify=off  T_priority=None  T=0 K  T_nominal_specify=off  T_nominal_unit=K  T_nominal_value=1
      settings: SourceProductBaseCode=PW,SS,VE
  A : PMIOPort  Side=Right
  connections:
  A/RConn1 -- Expansion Tank/RConn1
  Perfect Insulator2/LConn1 -- Expansion Tank/RConn2

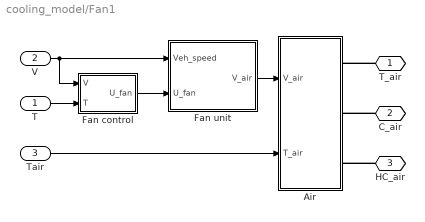
== system cooling_model/Fan1 ==
  T : Inport
  V : Inport  Port=2
  Tair : Inport  Port=3
  Air : Subsystem
  Fan control : Subsystem  mask(2-Level Fan Controller){T_level1=[97 94], T_level2=[105 102]}
      mask prompts: T_level1 "Level 1 temperature"; T_level2 "Level 2 temperature"
      mask help: The primary and secondary fan control temperature ranges are defined by Level 1 temperature vector and Level 2 temperature vector, respectively.
  Fan unit : Subsystem
  T_air : PMIOPort  Side=Right
  C_air : PMIOPort  Port=2  Side=Right
  HC_air : PMIOPort  Port=3  Side=Right
  wires:
  T/1 -> Fan control/2(T)
  Fan control/1(U_fan) -> Fan unit/2(U_fan)
  Fan unit/1(V_air) -> Air/1(V_air)
  V/1 -> Fan unit/1(Veh_speed), Fan control/1(V)
  Tair/1 -> Air/2(T_air)
  connections:
  HC_air/RConn1 -- Air/RConn3
  C_air/RConn1 -- Air/RConn2
  T_air/RConn1 -- Air/RConn1

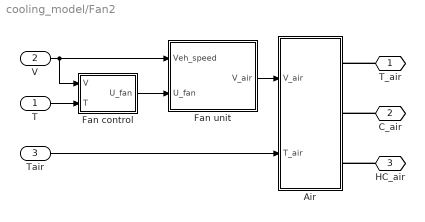
== system cooling_model/Fan2 ==
  T : Inport
  V : Inport  Port=2
  Tair : Inport  Port=3
  Air : Subsystem
  Fan control : Subsystem  mask(2-Level Fan Controller){T_level1=[97 94], T_level2=[105 102]}
      mask prompts: T_level1 "Level 1 temperature"; T_level2 "Level 2 temperature"
      mask help: The primary and secondary fan control temperature ranges are defined by Level 1 temperature vector and Level 2 temperature vector, respectively.
  Fan unit : Subsystem
  T_air : PMIOPort  Side=Right
  C_air : PMIOPort  Port=2  Side=Right
  HC_air : PMIOPort  Port=3  Side=Right
  wires:
  Tair/1 -> Air/2(T_air)
  V/1 -> Fan control/1(V), Fan unit/1(Veh_speed)
  Fan unit/1(V_air) -> Air/1(V_air)
  Fan control/1(U_fan) -> Fan unit/2(U_fan)
  T/1 -> Fan control/2(T)
  connections:
  T_air/RConn1 -- Air/RConn1
  C_air/RConn1 -- Air/RConn2
  HC_air/RConn1 -- Air/RConn3

== system cooling_model/Fan3 ==
  T : Inport
  V : Inport  Port=2
  Tair : Inport  Port=3
  Air : Subsystem
  Fan control : Subsystem  mask(2-Level Fan Controller){T_level1=[97 94], T_level2=[105 102]}
      mask prompts: T_level1 "Level 1 temperature"; T_level2 "Level 2 temperature"
      mask help: The primary and secondary fan control temperature ranges are defined by Level 1 temperature vector and Level 2 temperature vector, respectively.
  Fan unit : Subsystem
  T_air : PMIOPort  Side=Right
  C_air : PMIOPort  Port=2  Side=Right
  HC_air : PMIOPort  Port=3  Side=Right
  wires:
  T/1 -> Fan control/2(T)
  Fan control/1(U_fan) -> Fan unit/2(U_fan)
  Fan unit/1(V_air) -> Air/1(V_air)
  V/1 -> Fan unit/1(Veh_speed), Fan control/1(V)
  Tair/1 -> Air/2(T_air)
  connections:
  HC_air/RConn1 -- Air/RConn3
  C_air/RConn1 -- Air/RConn2
  T_air/RConn1 -- Air/RConn1

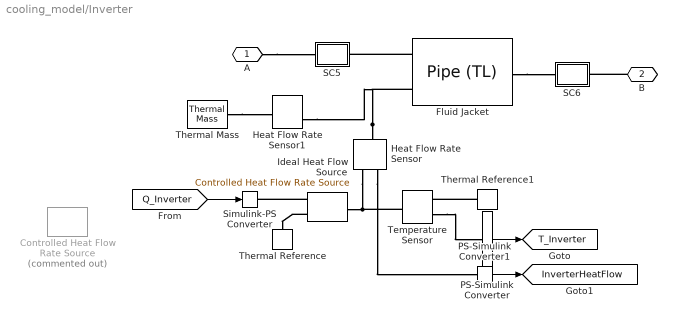
== system cooling_model/Inverter ==
  Controlled Heat Flow Rate Source : fl_lib/Thermal/Thermal Sources/Controlled Heat Flow Rate Source  Commented=on
      settings: SourceProductBaseCode=PW,SS,VE
  Fluid Jacket : SimscapeFluids_lib/Thermal Liquid/Pipes & Fittings/Pipe (TL)  dynamic_compressibility=simscape.enum.onoff.off  inertia=simscape.enum.onoff.off  num_segments=1  pipe_length=0.2 m  area=pi*0.01^2 m^2  wall_spec=fluids.thermal_liquid.pipes_fittings.enum.wall_spec.rigid  Dh=0.005 m  wall_compliance=1.2e-6 m/MPa  wall_time_constant=0.01 s  elevation_spec=foundation.enum.constant_variable.constant  elevation_gain=0 m  g=9.81 m/s^2  pressure_loss_spec=fluids.thermal_liquid.pipes_fittings.enum.PressureLossSpec.Nominal  local_pressure_loss_spec=fluids.thermal_liquid.pipes_fittings.enum.LocalLossSpec.AggregateLength  length_add=0 m  loss_coefficient=0.1  roughness=1.5e-60 m  Re_friction_TLU=[ 400 1000 1.5e+3 3e+3 4e+3 6e+3 1e+4 2e+4 4e+4 6e+4 1e+5 1e+8 ]  friction_factor_TLU=[ 0.264 0.112 0.07099999999999999 0.0417 0.0387 0.0268 0.025 0.0232 0.0226 0.022 0.0214 0.0214 ]  shape_factor=1e-50  Re_lam=2e+3  Re_tur=4e+3  mdot_nominal=[ 0.1 1000 ] kg/s  p_diff_nominal=[ 0.00000001 0.000000001 ] MPa  mdot_threshold=1e-6 kg/s  heat_transfer_spec=fluids.thermal_liquid.pipes_fittings.enum.HeatTransferSpec.TabulatedNusselt  mdot_nominal_heat=[ 0.1 1 ] kg/s  T_in_nominal=[ 293.15 293.15 ] K  T_out_nominal=[ 300 300 ] K  p_in_nominal_heat=[ 0.101325 0.101325 ] MPa  T_wall_nominal=[ 303.15 303.15 ] K  a_coeff=0.023  b_Re_power=0.8  c_Pr_power=0.4  Nu_lam=3.66  Re_Colburn_TLU=[ 100 150 1000 ]  Colburn_factor_TLU=[ 0.019 0.013 0.002 ]  Re_Nu_TLU=Re_TLU  Pr_Nu_TLU=Pr_TLU  Nu_TLU=Nu_TLU  T0_vec=303.15 K  p0_vec=0.101325 MPa  mdot0=0.1 kg/s
      settings: SourceProductBaseCode=SH
  Heat Flow Rate Sensor : fl_lib/Thermal/Thermal Sensors/Heat Flow Rate Sensor
      settings: SourceProductBaseCode=PW,SS,VE
  Heat Flow Rate Sensor1 : fl_lib/Thermal/Thermal Sensors/Heat Flow Rate Sensor
      settings: SourceProductBaseCode=PW,SS,VE
  Ideal Heat Flow Source : fl_lib/Thermal/Thermal Sources/Controlled Heat Flow Rate Source
      settings: SourceProductBaseCode=PW,SS,VE
  PS-Simulink Converter : nesl_utility/PS-Simulink Converter  PhysicalDomain=network_engine_domain  SubClassName=ps_output  LeftPortType=input  RightPortType=output  PseudoPeriodic=off  Frequencies=[]  VectorFormat=1-D array  Unit=degC  AffineConversion=on
      settings: SourceProductBaseCode=SS,PW,VE
  PS-Simulink Converter1 : nesl_utility/PS-Simulink Converter  PhysicalDomain=network_engine_domain  SubClassName=ps_output  LeftPortType=input  RightPortType=output  PseudoPeriodic=off  Frequencies=[]  VectorFormat=inherit  Unit=inherit  AffineConversion=off
      settings: SourceProductBaseCode=SS,PW,VE
  SC5 : Subsystem
      mask Display: disp(get_param(gcb, 'Name'))
  SC6 : Subsystem
      mask Display: disp(get_param(gcb, 'Name'))
  Simulink-PS Converter : nesl_utility/Simulink-PS Converter  PhysicalDomain=network_engine_domain  SubClassName=ps_input  LeftPortType=input  RightPortType=output  PseudoPeriodic=off  Frequencies=[]  NoiseDistribution=none  NoiseParameters=[]  Unit=W  AffineConversion=off  FilteringAndDerivatives=provide  SimscapeFilterOrder=1  InputFilterTimeConstant=0.001  UdotUserProvided=0
      settings: SourceProductBaseCode=SS,PW,VE
  Temperature Sensor : fl_lib/Thermal/Thermal Sensors/Temperature Sensor
      settings: SourceProductBaseCode=PW,SS,VE
  Thermal Mass : fl_lib/Thermal/Thermal Elements/Thermal Mass  mass=60 kg  sp_heat=447 J/(K*kg)  T_specify=on  T_priority=High  T=273+45 K  T_nominal_specify=on  T_nominal_unit=K  T_nominal_value=273.15+45  Q_specify=off  Q_priority=None  Q=0 W  Q_nominal_specify=off  Q_nominal_unit=W  Q_nominal_value=1
      settings: SourceProductBaseCode=PW,SS,VE
  Thermal Reference : fl_lib/Thermal/Thermal Elements/Thermal Reference
      settings: SourceProductBaseCode=PW,SS,VE
  Thermal Reference1 : fl_lib/Thermal/Thermal Elements/Thermal Reference
      settings: SourceProductBaseCode=PW,SS,VE
  A : PMIOPort  Side=Left
  B : PMIOPort  Port=2  Side=Right
  tag scope: InverterHeatFlow=global, T_Inverter=global
  wires:
  PS-Simulink Converter1/1 -> [InverterHeatFlow]
  PS-Simulink Converter/1 -> [T_Inverter]
  [Q_Inverter] -> Simulink-PS Converter/1
  connections:
  Thermal Mass/LConn1 -- Heat Flow Rate Sensor1/LConn1
  Fluid Jacket/RConn1 -- SC6/LConn1
  Fluid Jacket/LConn1 -- SC5/RConn1
  Heat Flow Rate Sensor/RConn1 -- PS-Simulink Converter1/LConn1
  Heat Flow Rate Sensor/LConn1 -- Heat Flow Rate Sensor1/RConn2 -- Fluid Jacket/LConn2
  Temperature Sensor/RConn2 -- PS-Simulink Converter/LConn1
  Thermal Reference1/LConn1 -- Temperature Sensor/RConn1
  Ideal Heat Flow Source/RConn1 -- Simulink-PS Converter/RConn1
  A/RConn1 -- SC5/LConn1
  Ideal Heat Flow Source/RConn2 -- Thermal Reference/LConn1
  B/RConn1 -- SC6/RConn1
  Ideal Heat Flow Source/LConn1 -- Heat Flow Rate Sensor/RConn2 -- Temperature Sensor/LConn1
